simulink subsystem "gimbal"  (R2022b)
settings: Solver=VariableStepAuto  StartTime=0.0  StopTime=10.0  RelTol=1e-3
values from neighbouring files (symbols this model uses):
  Ip = Ifz    (= 0.09)    [gyro_and_bicycle_params.m]
settings Model: Creator=baran  LastModifiedBy=baran

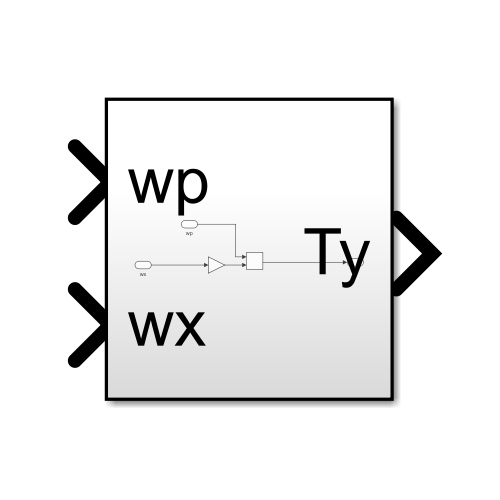
[thumbnail: Simulink's stored preview of the top-level diagram]
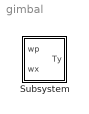
== system gimbal ==
  Subsystem : Subsystem

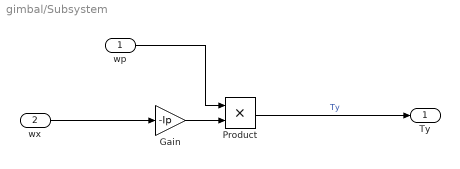
== system gimbal/Subsystem ==
  wp : Inport
  wx : Inport  Port=2
  Gain : Gain  Gain=-Ip
  Product : Product
  Ty : Outport
  wires:
  Gain/1 -> Product/2
  Product/1 -> Ty/1  "Ty"
  wx/1 -> Gain/1
  wp/1 -> Product/1
